simulink model "ai_optimal_path_depth_v2_3_g100"  (R2020a)
settings: Solver=FixedStepDiscrete  StartTime=0.0  StopTime=inf  FixedStep=0.2  RelTol=1e-3  EnableMultiTasking=on
model workspace (MAT data in the model file):
  SL_ROS_VariableLengthArrays_MaxSizes.CommonInfo.ArrayTruncateAction = 'EmitWarning'
  SL_ROS_VariableLengthArrays_MaxSizes.MsgTypeMap = containers.Map
  SL_ROS_VariableLengthArrays_MaxSizes.MsgTypeMap.serialization.keys = {'sensor_msgs/LaserScan', 'sensor_msgs/PointCloud2', 'std_msgs/Float64MultiArray'}
  SL_ROS_VariableLengthArrays_MaxSizes.MsgTypeMap.serialization.values{1}(1).PropertyName = 'Intensities'
  SL_ROS_VariableLengthArrays_MaxSizes.MsgTypeMap.serialization.values{1}(1).DataType = 'single'
  SL_ROS_VariableLengthArrays_MaxSizes.MsgTypeMap.serialization.values{1}(1).MaxLength = 360
  SL_ROS_VariableLengthArrays_MaxSizes.MsgTypeMap.serialization.values{1}(2).PropertyName = 'Ranges'
  SL_ROS_VariableLengthArrays_MaxSizes.MsgTypeMap.serialization.values{1}(2).DataType = 'single'
  SL_ROS_VariableLengthArrays_MaxSizes.MsgTypeMap.serialization.values{1}(2).MaxLength = 360
  SL_ROS_VariableLengthArrays_MaxSizes.MsgTypeMap.serialization.values{2}(1).PropertyName = 'Data'
  SL_ROS_VariableLengthArrays_MaxSizes.MsgTypeMap.serialization.values{2}(1).DataType = 'uint8'
  SL_ROS_VariableLengthArrays_MaxSizes.MsgTypeMap.serialization.values{2}(1).MaxLength = 600000
  SL_ROS_VariableLengthArrays_MaxSizes.MsgTypeMap.serialization.values{2}(2).PropertyName = 'Fields'
  SL_ROS_VariableLengthArrays_MaxSizes.MsgTypeMap.serialization.values{2}(2).DataType = 'sensor_msgs/PointField'
  SL_ROS_VariableLengthArrays_MaxSizes.MsgTypeMap.serialization.values{2}(2).MaxLength = 16
  SL_ROS_VariableLengthArrays_MaxSizes.MsgTypeMap.serialization.values{3}.PropertyName = 'Data'
  SL_ROS_VariableLengthArrays_MaxSizes.MsgTypeMap.serialization.values{3}.DataType = 'double'
  SL_ROS_VariableLengthArrays_MaxSizes.MsgTypeMap.serialization.values{3}.MaxLength = 360
  SL_ROS_VariableLengthArrays_MaxSizes.MsgTypeMap.serialization.uniformity = 0
  SL_ROS_VariableLengthArrays_MaxSizes.MsgTypeMap.serialization.keyType = 'char'
  SL_ROS_VariableLengthArrays_MaxSizes.MsgTypeMap.serialization.valueType = 'any'
undefined symbols (not defined in the file): Data, Data_SL_Info
libraries: robotlib x29
(part 1 of 2)
settings Model: Creator=USER  LastModifiedBy=USER
settings SolverCC: InsertRTBMode=Never (minimum delay)
settings DataIOCC: ReturnWorkspaceOutputs=off
settings OptimizationCC: StrengthReduction=on  PassReuseOutputArgsAs=Individual arguments  MaxStackSize=64  OptimizeBlockOrder=speed  OptimizationPriority=Speed  OptimizationCustomize=off  MultiThreadedLoops=on  EfficientTunableParamExpr=on
settings DebuggingCC: ParameterTunabilityLossMsg=error  PregeneratedLibrarySubsystemCodeDiagnostic=none  ArithmeticOperatorsInVariantConditions=warning
settings HardwareCC: ProdBitPerPointer=32  ProdBitPerSizeT=32  ProdBitPerPtrDiffT=32  ProdLargestAtomicFloat=None  ProdIntDivRoundTo=Undefined  ProdEndianess=Unspecified  ProdWordSize=32  ProdHWDeviceType=Generic->Unspecified (assume 32-bit Generic)
settings SFSimCC: SimUseLocalCustomCode=off  MATLABDynamicMemAlloc=off  CustomCodeUndefinedFunction=UseInterfaceOnly
settings RTWCC: SystemTargetFile=ert.tlc  HardwareBoard=Robot Operating System (ROS)  TemplateMakefile=ert_default_tmf  GenerateReport=on  RTWUseLocalCustomCode=off  Toolchain=Catkin  BuildConfiguration=Faster Runs  IncludeHyperlinkInReport=on  LaunchReport=on  TargetLang=C++  GenerateTraceInfo=on  GenerateTraceReport=on  GenerateTraceReportSl=on  GenerateTraceReportSf=on  GenerateTraceReportEml=on
settings CodeAppCC: ForceParamTrailComments=on  IgnoreCustomStorageClasses=off  OperatorAnnotations=on  SimulinkDataObjDesc=on  SFDataObjDesc=on  InsertBlockDesc=on
settings ERTTargetCC: SupportVariableSizeSignals=on

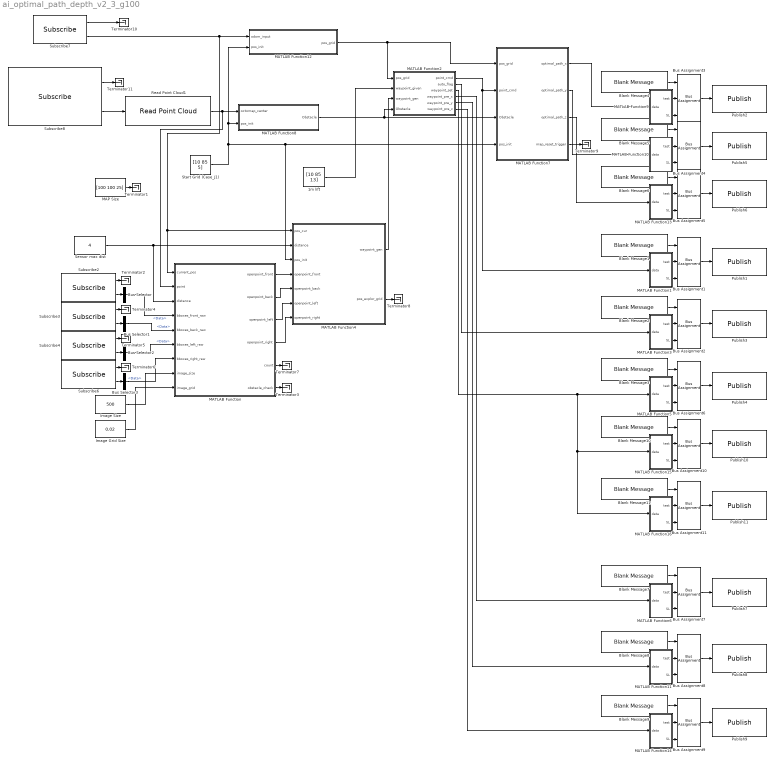
== system ai_optimal_path_depth_v2_3_g100 ==
  1m lift : Constant  Value=[10 85 13]  VectorParams1D=off
  Blank Message{1..11} (11 alike) : robotlib/Blank Message  messageClass=Message  entityType=std_msgs/Float32MultiArray  messageType=std_msgs/Float32MultiArray  SampleTime=-1
  Bus Assignment{1..11} (11 alike) : BusAssignment  AssignedSignals=Data,Data_SL_Info.CurrentLength
  Bus Selector{,1..3} (4 alike) : BusSelector  OutputSignals=Data
  Image Grid Size : Constant  Value=0.02
  Image Size : Constant  Value=500
  MAP Size : Constant  Value=[100 100 25]
  MATLAB Function : MATLAB Function  TreatAsAtomicUnit=on
  MATLAB Function1 : MATLAB Function  TreatAsAtomicUnit=on
  MATLAB Function10 : MATLAB Function  TreatAsAtomicUnit=on
  MATLAB Function11 : MATLAB Function  TreatAsAtomicUnit=on
  MATLAB Function12 : MATLAB Function  TreatAsAtomicUnit=on
  MATLAB Function13 : MATLAB Function  TreatAsAtomicUnit=on
  MATLAB Function14 : MATLAB Function  TreatAsAtomicUnit=on
  MATLAB Function15 : MATLAB Function  TreatAsAtomicUnit=on
  MATLAB Function16 : MATLAB Function  TreatAsAtomicUnit=on
  MATLAB Function2 : MATLAB Function  TreatAsAtomicUnit=on
  MATLAB Function3 : MATLAB Function  TreatAsAtomicUnit=on
  MATLAB Function4 : MATLAB Function  TreatAsAtomicUnit=on
  MATLAB Function5 : MATLAB Function  TreatAsAtomicUnit=on
  MATLAB Function6 : MATLAB Function  TreatAsAtomicUnit=on
  MATLAB Function7 : MATLAB Function  TreatAsAtomicUnit=on
  MATLAB Function8 : MATLAB Function  TreatAsAtomicUnit=on
  MATLAB Function9 : MATLAB Function  TreatAsAtomicUnit=on
  Publish1 : robotlib/Publish  topicSource=Specify your own  topic=/current_point_cmd  messageType=std_msgs/Float32MultiArray  messageQueueLength=1
  Publish10 : robotlib/Publish  topicSource=Specify your own  topic=/waypoint_set_y  messageType=std_msgs/Float32MultiArray  messageQueueLength=1
  Publish11 : robotlib/Publish  topicSource=Specify your own  topic=/waypoint_set_z  messageType=std_msgs/Float32MultiArray  messageQueueLength=1
  Publish2 : robotlib/Publish  topicSource=Specify your own  topic=/optimal_path_x  messageType=std_msgs/Float32MultiArray  messageQueueLength=1
  Publish3 : robotlib/Publish  topicSource=Specify your own  topic=/auto_flag  messageType=std_msgs/Float32MultiArray  messageQueueLength=1
  Publish4 : robotlib/Publish  topicSource=Specify your own  topic=/waypoint_set_x  messageType=std_msgs/Float32MultiArray  messageQueueLength=1
  Publish5 : robotlib/Publish  topicSource=Specify your own  topic=/optimal_path_y  messageType=std_msgs/Float32MultiArray  messageQueueLength=1
  Publish6 : robotlib/Publish  topicSource=Specify your own  topic=/optimal_path_z  messageType=std_msgs/Float32MultiArray  messageQueueLength=1
  Publish7 : robotlib/Publish  topicSource=Specify your own  topic=/waypoint_pre_x  messageType=std_msgs/Float32MultiArray  messageQueueLength=1
  Publish8 : robotlib/Publish  topicSource=Specify your own  topic=/waypoint_pre_y  messageType=std_msgs/Float32MultiArray  messageQueueLength=1
  Publish9 : robotlib/Publish  topicSource=Specify your own  topic=/waypoint_pre_z  messageType=std_msgs/Float32MultiArray  messageQueueLength=1
  Read Point Cloud1 : robotlib/Read Point Cloud  MaximumPointCloudSize=[1, 650000]  PreserveStructure=off  ShowRGBOutput=off  ShowIntensityOutput=off  ShowErrorCodeOutput=off  VariableSizeOutputs=on
      settings: SourceProductBaseCode=RR
  Sensor max dist : Constant  Value=4
  Start Grid (Case_J1) : Constant  Value=[10 85 5]
  Subscribe2 : robotlib/Subscribe  topicSource=Select from ROS network  topic=/bboxes_front  messageType=std_msgs/Float32MultiArray  sampleTime=-1  messageQueueLength=1
  Subscribe3 : robotlib/Subscribe  topicSource=Select from ROS network  topic=/bboxes_back  messageType=std_msgs/Float32MultiArray  sampleTime=-1  messageQueueLength=1
  Subscribe4 : robotlib/Subscribe  topicSource=Select from ROS network  topic=/bboxes_left  messageType=std_msgs/Float32MultiArray  sampleTime=-1  messageQueueLength=1
  Subscribe6 : robotlib/Subscribe  topicSource=Select from ROS network  topic=/bboxes_right  messageType=std_msgs/Float32MultiArray  sampleTime=-1  messageQueueLength=1
  Subscribe7 : robotlib/Subscribe  topicSource=Select from ROS network  topic=/rtabmap/odom  messageType=nav_msgs/Odometry  sampleTime=-1  messageQueueLength=1
  Subscribe8 : robotlib/Subscribe  topicSource=Select from ROS network  topic=/rtabmap/cloud_map  messageType=sensor_msgs/PointCloud2  sampleTime=-1  messageQueueLength=1
  Terminator{1..11} (11 alike) : Terminator
  wires:
  MATLAB Function9/1(test) -> Bus Assignment3/2
  Blank Message4/1 -> Bus Assignment3/1
  Bus Assignment4/1 -> Publish5/1
  Blank Message5/1 -> Bus Assignment4/1
  MATLAB Function9/2(SL) -> Bus Assignment3/3
  Subscribe7/2 -> MATLAB Function4/1(pos_cur), MATLAB Function/1(current_pos), MATLAB Function12/1(odom_input)
  MATLAB Function13/2(SL) -> Bus Assignment5/3
  Start Grid (Case_J1)/1 -> MATLAB Function4/3(pos_init), MATLAB Function7/4(pos_init), MATLAB Function8/2(pos_init), MATLAB Function12/2(pos_init)
  MATLAB Function12/1(pos_grid) -> MATLAB Function7/1(pos_grid), MATLAB Function2/1(pos_grid)
  MATLAB Function10/1(test) -> Bus Assignment4/2
  MATLAB Function13/1(test) -> Bus Assignment5/2
  Bus Assignment5/1 -> Publish6/1
  MATLAB Function10/2(SL) -> Bus Assignment4/3
  Blank Message6/1 -> Bus Assignment5/1
  Bus Assignment3/1 -> Publish2/1
  MAP Size/1 -> Terminator1/1
  MATLAB Function8/1(Obstacle) -> MATLAB Function7/3(Obstacle), MATLAB Function2/4(Obstacle)
  MATLAB Function7/1(optimal_path_x) -> MATLAB Function9/1(data)
  MATLAB Function7/2(optimal_path_y) -> MATLAB Function10/1(data)
  MATLAB Function7/3(optimal_path_z) -> MATLAB Function13/1(data)
  1m lift/1 -> MATLAB Function2/2(waypoint_given)
  Read Point Cloud1/1 -> MATLAB Function/2(point), MATLAB Function8/1(octomap_center)
  Subscribe8/2 -> Read Point Cloud1/1
  MATLAB Function2/1(point_cmd) -> MATLAB Function7/2(point_cmd), MATLAB Function1/1(data)
  Subscribe2/1 -> Terminator2/1
  Subscribe3/1 -> Terminator4/1
  Subscribe4/1 -> Terminator5/1
  Subscribe6/1 -> Terminator6/1
  Subscribe2/2 -> Bus Selector/1
  Subscribe3/2 -> Bus Selector1/1
  Subscribe4/2 -> Bus Selector2/1
  Subscribe6/2 -> Bus Selector3/1
  Image Size/1 -> MATLAB Function/8(image_size)
  Image Grid Size/1 -> MATLAB Function/9(image_grid)
  Sensor max dist/1 -> MATLAB Function4/2(distance), MATLAB Function/3(distance)
  MATLAB Function/1(openpoint_front) -> MATLAB Function4/4(openpoint_front)
  MATLAB Function/2(openpoint_back) -> MATLAB Function4/5(openpoint_back)
  MATLAB Function/3(openpoint_left) -> MATLAB Function4/6(openpoint_left)
  MATLAB Function/4(openpoint_right) -> MATLAB Function4/7(openpoint_right)
  MATLAB Function/5(count) -> Terminator7/1
  MATLAB Function4/2(pos_explor_grid) -> Terminator8/1
  Bus Selector/1 -> MATLAB Function/4(bboxes_front_raw)  "<Data>"
  Bus Selector1/1 -> MATLAB Function/5(bboxes_back_raw)  "<Data>"
  Bus Selector2/1 -> MATLAB Function/6(bboxes_left_raw)  "<Data>"
  Bus Selector3/1 -> MATLAB Function/7(bboxes_right_raw)  "<Data>"
  MATLAB Function7/4(map_reset_trigger) -> Terminator9/1
  MATLAB Function4/1(waypoint_gen) -> MATLAB Function2/3(waypoint_gen)
  MATLAB Function2/2(auto_flag) -> MATLAB Function3/1(data)
  MATLAB Function2/3(waypoint_set) -> MATLAB Function16/1(data), MATLAB Function15/1(data), MATLAB Function5/1(data)
  MATLAB Function1/1(test) -> Bus Assignment1/2
  Bus Assignment1/1 -> Publish1/1
  MATLAB Function1/2(SL) -> Bus Assignment1/3
  Blank Message1/1 -> Bus Assignment1/1
  Blank Message2/1 -> Bus Assignment2/1
  MATLAB Function3/2(SL) -> Bus Assignment2/3
  MATLAB Function3/1(test) -> Bus Assignment2/2
  Bus Assignment2/1 -> Publish3/1
  Blank Message3/1 -> Bus Assignment6/1
  MATLAB Function5/2(SL) -> Bus Assignment6/3
  MATLAB Function5/1(test) -> Bus Assignment6/2
  Bus Assignment6/1 -> Publish4/1
  MATLAB Function6/2(SL) -> Bus Assignment7/3
  MATLAB Function6/1(test) -> Bus Assignment7/2
  Blank Message7/1 -> Bus Assignment7/1
  Bus Assignment7/1 -> Publish7/1
  MATLAB Function11/1(test) -> Bus Assignment8/2
  Bus Assignment8/1 -> Publish8/1
  MATLAB Function11/2(SL) -> Bus Assignment8/3
  Blank Message8/1 -> Bus Assignment8/1
  MATLAB Function14/1(test) -> Bus Assignment9/2
  Bus Assignment9/1 -> Publish9/1
  MATLAB Function14/2(SL) -> Bus Assignment9/3
  Blank Message9/1 -> Bus Assignment9/1
  MATLAB Function2/4(waypoint_pre_x) -> MATLAB Function6/1(data)
  MATLAB Function2/5(waypoint_pre_y) -> MATLAB Function11/1(data)
  MATLAB Function2/6(waypoint_pre_z) -> MATLAB Function14/1(data)
  Subscribe7/1 -> Terminator10/1
  Subscribe8/1 -> Terminator11/1
  MATLAB Function15/1(test) -> Bus Assignment10/2
  Blank Message10/1 -> Bus Assignment10/1
  MATLAB Function15/2(SL) -> Bus Assignment10/3
  Bus Assignment10/1 -> Publish10/1
  MATLAB Function16/1(test) -> Bus Assignment11/2
  Blank Message11/1 -> Bus Assignment11/1
  MATLAB Function16/2(SL) -> Bus Assignment11/3
  Bus Assignment11/1 -> Publish11/1
  MATLAB Function/6(obstacle_check) -> Terminator3/1

== matlab function ai_optimal_path_depth_v2_3_g100/MATLAB Function10 ==
  data: data input size=[128 1]; test output size=[1 128]; SL output
function [test,SL]   = func(data)

% test = single(nan(1,128));

test = data';
% for i = 1:length(data)
%     test(i) = single(data(i));
% end

SL = uint32(length(data));


end

== matlab function ai_optimal_path_depth_v2_3_g100/MATLAB Function11 ==
  data: data input size=[20 1]; test output size=[1 128]; SL output
function [test,SL]   = func(data)

% test = single(nan(1,128));

test = single([data(:,1)', nan(1,108)]);
% for i = 1:length(data)
%     test(i) = single(data(i));
% end

SL = uint32(length(data(:,1)));


end

== matlab function ai_optimal_path_depth_v2_3_g100/MATLAB Function12 ==
  data: odom_input input; pos_grid output; pos_init input
function pos_grid = odom_grid(odom_input,pos_init)

odom = zeros(1,3);


% odom(1,1) = odom_input.Poses(end).Pose.Position.X;
% odom(1,2) = odom_input.Poses(end).Pose.Position.Y;
% odom(1,3) = odom_input.Poses(end).Pose.Position.Z;

odom(1,1) = odom_input.Pose.Pose.Position.X;
odom(1,2) = odom_input.Pose.Pose.Position.Y;
odom(1,3) = odom_input.Pose.Pose.Position.Z;

start_point = [pos_init(1) pos_init(2) pos_init(3)];

% pos_x = int16(odom(1)/0.2+0.5);
% pos_y = int16(odom(2)/0.2+0.5);
% pos_z = int16(odom(3)/0.2+0.5);
pos_x = int16(odom(1)/0.1);
pos_y = int16(odom(2)/0.1);
pos_z = int16(odom(3)/0.1);

pos_grid = [pos_x+start_point(1) pos_y+start_point(2) pos_z+start_point(3)];


end

== matlab function ai_optimal_path_depth_v2_3_g100/MATLAB Function13 ==
  data: data input size=[128 1]; test output size=[1 128]; SL output
function [test,SL]   = func(data)


% test = single(nan(1,128));

test = data';
% for i = 1:length(data)
%     test(i) = single(data(i));
% end

SL = uint32(length(data));

end

== matlab function ai_optimal_path_depth_v2_3_g100/MATLAB Function7 ==
  data: pos_grid input; optimal_path_x output size=[128 1]; point_cmd input; Obstacle input; pos_init input; optimal_path_y output size=[128 1]; optimal_path_z output size=[128 1]; map_reset_trigger output
function [optimal_path_x,optimal_path_y,optimal_path_z,map_reset_trigger] = Astar_algorithm_function(pos_grid,point_cmd,Obstacle,pos_init)

    persistent optimal astar_restart curr_point hover_flag 

    if isempty(optimal)
        optimal = nan(128,3);
        hover_flag = 0;
        astar_restart = 1;
        curr_point = point_cmd;        
    end

    map_reset_trigger = 0;
    grid_size = 0.1;

    if (curr_point(1) ~= point_cmd(1)) || (curr_point(2) ~= point_cmd(2)) || (curr_point(3) ~= point_cmd(3))
        astar_restart = 1;
    end
    curr_point = point_cmd;
    
    if Obstacle(pos_grid(1), pos_grid(2), pos_grid(3)) == 1
        astar_restart = 0;
    end
    
    
%---------------------------------------------------------
% A* 시작
%---------------------------------------------------------
    if astar_restart == 1
        % ----------------------------------------------------- initilize
        astar_restart = 0;
        mapsize = [140 120 30];
        
        Height = mapsize(1);        % x
        Width = mapsize(2);         % y
        Alt = mapsize(3);            % z
        
        Start = pos_grid;
%         Goal = int32(point_cmd/grid_size + pos_init');          % 수정 
        Goal = int32(point_cmd);          % 수정 
        look = 2;
        H_weight = 1.3;
        
        G_cost = zeros(2*look+1,2*look+1,2*look+1);
        for i = 1:2*look+1
            for j = 1:2*look+1
                for k = 1:2*look+1
                    temp = [look+1 look+1 look+1]-[i j k];
                    G_cost(i,j,k) = (min(sqrt(sum(abs(temp).^2,2))));
                end
            end
        end
        
        G_top2 = G_cost(:,:,1);
        G_top1 = G_cost(:,:,2);
        G_mid = G_cost(:,:,3);
        G_bottom1 = G_cost(:,:,4);
        G_bottom2 = G_cost(:,:,5);
        
        
        GScore = inf(Height,Width,Alt);
        GScore_temp = zeros(2*look+1,2*look+1,2*look+1);
        HScore = zeros(Height,Width,Alt);
        FScore = inf(Height,Width,Alt);
        ClosedMAT = zeros(Height,Width,Alt);
        CX = int32(Start(1));
        CY = int32(Start(2));
        CZ = int32(Start(3));
        ParentX = inf(Height,Width,Alt);
        ParentY = inf(Height,Width,Alt);
        ParentZ = inf(Height,Width,Alt);
        ParentX(CX,CY,CZ) = CX;
        ParentY(CX,CY,CZ) = CY;
        ParentZ(CX,CY,CZ) = CZ;
        hover_flag = 0;
        
        %%%%%%%%%%%%%%%% Define Heuristic %%%%%%%%%%%%%%%%%%%%%%%
        for k=1:Alt
            for j=1:Width
                for i=1:Height
                    
                    temp = (int32(Goal) - int32([i j k])) ;
                    Distance=(min(sqrt(sum(abs(temp).^2,2))));
                    HScore(i,j,k)=Distance*H_weight;               % (1+sqrt(2))/sqrt(3)
                    
                end
            end
        end
        
        FScore(Start(1),Start(2),Start(3)) = HScore(Start(1),Start(2),Start(3));
        GScore(Start(1),Start(2),Start(3)) = 0;
        ClosedMAT(Obstacle==1)=1;
        REACHGOAL = 0;
        
        while 1
            fprintf("A* loop \n");
            MinFScore = min(min(min(FScore)));         % Find Minimun FScore
            
            if isinf(MinFScore)
                hover_flag = 1;
                astar_restart = 1;
                map_reset_trigger = 1;
                fprintf("No path -> restart A*, Map reset \n");
                break
            end
            
            [minF_x,minF_y] = find(FScore==MinFScore);
            HScore_temp = inf(1,10);
            
            minHScore = 1;
            for i = 1:length(minF_x)
                Current_pose_temp = [minF_x(i) rem(minF_y(i),Width) fix(minF_y(i)/Width)+1];     % H가 가장 적은걸로 먼저 선택
                CX_temp=Current_pose_temp(1);
                CY_temp=Current_pose_temp(2);
                CZ_temp=Current_pose_temp(3);
                HScore_temp(i) = HScore(CX_temp,CY_temp,CZ_temp);
                minHScore = find(HScore_temp == min(HScore_temp));
            end
            
            Current_pose = int32([minF_x(minHScore(1)) rem(minF_y(minHScore(1)),Width) fix(minF_y(minHScore(1))/Width)+1]);     % H가 가장 적은걸로 먼저 선택
            CX=Current_pose(1);
            CY=Current_pose(2);
            CZ=Current_pose(3);

            GScore_temp(:,:,1) = GScore(CX,CY,CZ) + G_top2;
            GScore_temp(:,:,2) = GScore(CX,CY,CZ) + G_top1;
            GScore_temp(:,:,3) = GScore(CX,CY,CZ) + G_mid;
            GScore_temp(:,:,4) = GScore(CX,CY,CZ) + G_bottom1;
            GScore_temp(:,:,5) = GScore(CX,CY,CZ) + G_bottom2;
            
            %%%%%%%%%%%%% GScore update %%%%%%%%%%%%%
            GScore(CX-look:CX+look,CY-look:CY+look,CZ+2) = min(GScore_temp(:,:,1),GScore(CX-look:CX+look,CY-look:CY+look,CZ+2)) ;
            GScore(CX-look:CX+look,CY-look:CY+look,CZ+1) = min(GScore_temp(:,:,2),GScore(CX-look:CX+look,CY-look:CY+look,CZ+1));
            GScore(CX-look:CX+look,CY-look:CY+look,CZ) = min(GScore_temp(:,:,3), GScore(CX-look:CX+look,CY-look:CY+look,CZ));
            GScore(CX-look:CX+look,CY-look:CY+look,CZ-1) = min(GScore_temp(:,:,4),GScore(CX-look:CX+look,CY-look:CY+look,CZ-1));
            GScore(CX-look:CX+look,CY-look:CY+look,CZ-2) = min(GScore_temp(:,:,5),GScore(CX-look:CX+look,CY-look:CY+look,CZ-2));
            
            FScore = GScore + HScore;
            ClosedMAT(CX-(look-1):CX+(look-1),CY-(look-1):CY+(look-1),CZ-(look-1):CZ+(look-1)) = 1;
            FScore(ClosedMAT==1) = inf;
            
            [G_row1,G_col1] = find( GScore(CX-look:CX+look,CY-look:CY+look,CZ+2) == GScore_temp(:,:,1) );
            [G_row2,G_col2] = find( GScore(CX-look:CX+look,CY-look:CY+look,CZ+1) == GScore_temp(:,:,2) );
            [G_row3,G_col3] = find( GScore(CX-look:CX+look,CY-look:CY+look,CZ) == GScore_temp(:,:,3) );
            [G_row4,G_col4] = find( GScore(CX-look:CX+look,CY-look:CY+look,CZ-1) == GScore_temp(:,:,4) );
            [G_row5,G_col5] = find( GScore(CX-look:CX+look,CY-look:CY+look,CZ-2) == GScore_temp(:,:,5) );
            
            G_row1 = int32(G_row1);
            G_row2 = int32(G_row2);
            G_row3 = int32(G_row3);
            G_row4 = int32(G_row4);
            G_row5 = int32(G_row5);
            
            G_col1 = int32(G_col1);
            G_col2 = int32(G_col2);
            G_col3 = int32(G_col3);
            G_col4 = int32(G_col4);
            G_col5 = int32(G_col5);
            
            G_row1 = G_row1+CX-(look+1);
            G_row2 = G_row2+CX-(look+1);
            G_row3 = G_row3+CX-(look+1);
            G_row4 = G_row4+CX-(look+1);
            G_row5 = G_row5+CX-(look+1);
            
            G_col1 = G_col1+CY-(look+1);
            G_col2 = G_col2+CY-(look+1);
            G_col3 = G_col3+CY-(look+1);
            G_col4 = G_col4+CY-(look+1);
            G_col5 = G_col5+CY-(look+1);
            
            for i = 1:length(G_row1)
                ParentX(G_row1(i),G_col1(i),CZ+2) = CX;
                ParentY(G_row1(i),G_col1(i),CZ+2) = CY;
                ParentZ(G_row1(i),G_col1(i),CZ+2) = CZ;
            end
            
            for i = 1:length(G_row2)
                ParentX(G_row2(i),G_col2(i),CZ+1) = CX;
                ParentY(G_row2(i),G_col2(i),CZ+1) = CY;
                ParentZ(G_row2(i),G_col2(i),CZ+1) = CZ;
            end
            
            for i = 1:length(G_row3)
                if G_row3(i)==CX && G_col3(i)==CY
                    continue
                end
                ParentX(G_row3(i),G_col3(i),CZ) = CX;
                ParentY(G_row3(i),G_col3(i),CZ) = CY;
                ParentZ(G_row3(i),G_col3(i),CZ) = CZ;
            end
            
            for i = 1:length(G_row4)
                ParentX(G_row4(i),G_col4(i),CZ-1) = CX;
                ParentY(G_row4(i),G_col4(i),CZ-1) = CY;
                ParentZ(G_row4(i),G_col4(i),CZ-1) = CZ;
            end
            
            for i = 1:length(G_row5)
                ParentX(G_row5(i),G_col5(i),CZ-2) = CX;
                ParentY(G_row5(i),G_col5(i),CZ-2) = CY;
                ParentZ(G_row5(i),G_col5(i),CZ-2) = CZ;
            end
            
            if abs(Goal(1)-CX)<=(look-1) && abs(Goal(2)-CY)<=(look-1) && abs(Goal(3)-CZ)<=(look-1)
                REACHGOAL = 1;
                fprintf("path founded\n");
                break
            end
        end
        
        optimal = nan(128,3);
        if REACHGOAL
            optimal(1,:) = [Goal(1) Goal(2) Goal(3)];
            k=2;
            while 1
                CX_temp = int32(ParentX(CX,CY,CZ));
                CY_temp = int32(ParentY(CX,CY,CZ));
                CZ_temp = int32(ParentZ(CX,CY,CZ));
                
                CX = CX_temp;
                CY = CY_temp;
                CZ = CZ_temp;
                
                optimal(k,:) = [CX CY CZ];
                k = k+1;
                
                if CX==Start(1) && CY==Start(2) && CZ==Start(3)
                    break
                end
            end
        end
        
    end
    
    if hover_flag == 0
            nan_check = isnan(optimal(:,1));
            for i = 1:1:128
                if nan_check(i) == 0
                    %fprintf("i:%d (%d,%d,%d) %d    ", int32(i), int32(optimal(i,1)), int32(optimal(i,2)), int32(optimal(i,3)), int32(Obstacle(optimal(i,1), optimal(i,2), optimal(i,3))));
                    if Obstacle(optimal(i,1), optimal(i,2), optimal(i,3)) == 1
                        astar_restart = 1;
                        fprintf("path collision! \n");
                        break;
                    end
                    %fprintf("not break \n");
                end
                astar_restart = 0;
            end
            % fprintf("collision check done \n");
    end
        
    if hover_flag == 1
        fprintf("hover flag on \n");
        hover_point = nan(128,3);
        hover_point(1,:) = [pos_grid(1) pos_grid(2) pos_grid(3)];
        optimal_path_x = flip(single( (hover_point(:,1)-pos_init(1)) * grid_size ));      % grid_size = 0.2,
        optimal_path_y = flip(single( (hover_point(:,2)-pos_init(2)) * grid_size ));
        optimal_path_z = flip(single( (hover_point(:,3)-pos_init(3)) * grid_size ));
    else
        optimal_path_x = flip(single( (optimal(:,1)-pos_init(1)) * grid_size ));      % grid_size = 0.2
        optimal_path_y = flip(single( (optimal(:,2)-pos_init(2)) * grid_size ));
        optimal_path_z = flip(single( (optimal(:,3)-pos_init(3)) * grid_size ));
    end
    
    
end

== matlab function ai_optimal_path_depth_v2_3_g100/MATLAB Function8 ==
  data: octomap_center input size=[650000 3]; Obstacle output size=[140 120 30]; pos_init input
function Obstacle = gen_3d_array(octomap_center,pos_init)
mapsize=[140 120 30];
Obstacle = int8(zeros(mapsize(1),mapsize(2),mapsize(3)));
start_point = [pos_init(1) pos_init(2) pos_init(3)];

grid_size = 0.1;
drone_size_xy = 0.2; % m
safety_size_xy = 0.2; % m
drone_size_z = 0.1; % m
safety_size_z = 0.1; % m
scattering_cells_xy = ceil((drone_size_xy + safety_size_xy)/grid_size);
scattering_cells_z = ceil((drone_size_z + safety_size_z)/grid_size);

test=[scattering_cells_xy+1 scattering_cells_xy+1 scattering_cells_z+1];

scattering_array = int8(zeros(scattering_cells_xy*2+1, scattering_cells_xy*2+1, scattering_cells_z*2+1));
for i=0:scattering_cells_xy
    for j=0:scattering_cells_xy
        if i^2+j^2 <= ((drone_size_xy + safety_size_xy)/grid_size)^2 
            scattering_array(i+test(1), j+test(2), -scattering_cells_z+test(3):scattering_cells_z + test(3)) = 1;
            scattering_array(i+test(1), -j+test(2), -scattering_cells_z+test(3):scattering_cells_z + test(3)) = 1;
            scattering_array(-i+test(1), j+test(2), -scattering_cells_z+test(3):scattering_cells_z + test(3)) = 1;
            scattering_array(-i+test(1), -j+test(2), -scattering_cells_z+test(3):scattering_cells_z + test(3)) = 1;
        end
    end
end
% scattering_array

align1 = int16(octomap_center/(grid_size));
align2 = unique(align1,'rows');
align3 = [align2(:,1)+start_point(1) align2(:,2)+start_point(2) align2(:,3)+start_point(3)]; % for ROS axis
%align3 = [align2(:,2)+start_point(1) -align2(:,1)+start_point(2) align2(:,3)+start_point(3)]; % for Fiesta axis

for i = 1:numel(align3)/3
    
    index_temp = align3(i,:);

    for j=1:scattering_cells_xy*2+1
        if index_temp(1)+j-1 - scattering_cells_xy <= 0 || index_temp(1)+j-1 - scattering_cells_xy > mapsize(1)
            continue;
        end    
        for k=1:scattering_cells_xy*2+1
            if index_temp(2)+k-1 -scattering_cells_xy <= 0 || index_temp(2)+k-1 - scattering_cells_xy > mapsize(2)
                continue;
            end
            for l=1:scattering_cells_z*2+1
                if index_temp(3)+l-1 - scattering_cells_z <= 0 || index_temp(3)+l-1 - scattering_cells_z > mapsize(3)
                    continue;
                end
                if scattering_array(j, k, l) == 1
                    Obstacle(index_temp(1)+j-1-scattering_cells_xy, index_temp(2)+k-1-scattering_cells_xy, index_temp(3)+l-1-scattering_cells_z) = 1;
                end
            end

        end
    end
end

Obstacle(1:3,:,:)=1;
Obstacle(mapsize(1)-2:mapsize(1),:,:) = 1;
Obstacle(:,1:3,:) = 1;
Obstacle(:,mapsize(2)-2:mapsize(2),:) = 1;
Obstacle(:,:,1:4) = 1;
Obstacle(:,:,mapsize(3)-10:mapsize(3)) = 1; % 고도제한 1.5m 

end

== matlab function ai_optimal_path_depth_v2_3_g100/MATLAB Function9 ==
  data: data input size=[128 1]; test output size=[1 128]; SL output
function [test,SL]   = func(data)

% test = single(nan(1,128));

test = data';
% for i = 1:length(data)
%     test(i) = single(data(i));
% end

SL = uint32(length(data));


end

== matlab function ai_optimal_path_depth_v2_3_g100/MATLAB Function14 ==
  data: data input size=[20 1]; test output size=[1 128]; SL output
function [test,SL]   = func(data)

% test = single(nan(1,128));

test = single([data(:,1)', nan(1,108)]);
% for i = 1:length(data)
%     test(i) = single(data(i));
% end

SL = uint32(length(data(:,1)));


end

== matlab function ai_optimal_path_depth_v2_3_g100/MATLAB Function15 ==
  data: data input size=[40 3]; test output size=[1 128]; SL output
function [test,SL]   = func(data)

% test = single(nan(1,128));

test = single([data(:,2)', nan(1,88)]);
% for i = 1:length(data)
%     test(i) = single(data(i));
% end

SL = uint32(length(data(:,2)));


end

== matlab function ai_optimal_path_depth_v2_3_g100/MATLAB Function16 ==
  data: data input size=[40 3]; test output size=[1 128]; SL output
function [test,SL]   = func(data)

% test = single(nan(1,128));

test = single([data(:,3)', nan(1,88)]);
% for i = 1:length(data)
%     test(i) = single(data(i));
% end

SL = uint32(length(data(:,3)));


end

== matlab function ai_optimal_path_depth_v2_3_g100/MATLAB Function1 ==
  data: data input size=[1 3]; test output size=[1 128]; SL output
function [test,SL]   = func(data)
% function [test,SL]   = func(data,pos_init)

% test = single(nan(1,128));

% test = single([single(data)-single(pos_init'), nan(1,125)])*0.2;
test = single([data, nan(1,125)]);
% for i = 1:length(data)
%     test(i) = single(data(i));
% end

SL = uint32(length(data));


end

== matlab function ai_optimal_path_depth_v2_3_g100/MATLAB Function2 ==
  data: pos_grid input; point_cmd output; waypoint_given input; waypoint_gen input; Obstacle input; auto_flag output; waypoint_set output; waypoint_pre_x output; waypoint_pre_y output; waypoint_pre_z output
function [point_cmd,auto_flag,waypoint_set,waypoint_pre_x,waypoint_pre_y,waypoint_pre_z] = gen_waypoint(pos_grid,waypoint_given,waypoint_gen,Obstacle)

persistent flag autonomous_mode_flag waypoint_old waypoint_pre

if isempty(flag)
    flag = 1;
end
if isempty(autonomous_mode_flag)
    autonomous_mode_flag = 0;
%     autonomous_mode_flag = 1;
end
if isempty(waypoint_old)
    waypoint_old = nan(20,3);
end
% num_waypoint_given = numel(waypoint_given)/3;
num_waypoint_given = 1;
if isempty(waypoint_pre)
    waypoint_pre = nan(20,3);
    for aaa = 1:num_waypoint_given
        waypoint_pre(aaa,1)=waypoint_given(aaa,1);
        waypoint_pre(aaa,2)=waypoint_given(aaa,2);
        waypoint_pre(aaa,3)=waypoint_given(aaa,3);
    end
end

pos_grid = int32(pos_grid);

waypoint_pre_x = waypoint_pre(:,1);
waypoint_pre_y = waypoint_pre(:,2);
waypoint_pre_z = waypoint_pre(:,3);

point_cmd_temp = int32([waypoint_pre_x(flag) waypoint_pre_y(flag) waypoint_pre_z(flag)]);
waypoint_gen_sorted = nan(20,3);
waypoint_auto_set = nan(40,3);
waypoint_auto_set_sorted = nan(40,3);
waypoint_distance = nan(40,1);

for lll = 1:numel(waypoint_gen)/3
    if ~isnan(waypoint_gen(lll,1)) && ~isnan(waypoint_gen(lll,2)) && ~isnan(waypoint_gen(lll,3))
        if Obstacle(waypoint_gen(lll,1),waypoint_gen(lll,2),waypoint_gen(lll,3)) == 1
            waypoint_gen(lll,:)=nan(1,3);
        end
    end
end


if autonomous_mode_flag==0
    if abs(point_cmd_temp(1)-pos_grid(1)) <= 1 && abs(point_cmd_temp(2)-pos_grid(2)) <= 1 && abs(point_cmd_temp(3)-pos_grid(3)) <= 1
        flag = flag + 1;
        
        %         if flag == numel(rmmissing(waypoint_pre))/3 + 1
        %             flag = numel(rmmissing(waypoint_pre))/3;
%         if flag == num_waypoint_given + 1
        if flag > num_waypoint_given
            flag = num_waypoint_given;
            autonomous_mode_flag = 1;
        end
    end
    
elseif autonomous_mode_flag==1
    %     waypoint_auto_old = rmmissing(waypoint_old);
    %     waypoint_auto_new = rmmissing(waypoint_gen);
    
    
    waypoint_auto_old = waypoint_old;
    [~,waypoint_gen_index]=sort(waypoint_gen(:,1));
    for aaa = 1:length(waypoint_gen_index)
        waypoint_gen_sorted(aaa,:)=waypoint_gen(waypoint_gen_index(aaa),:);
    end
    waypoint_auto_new=waypoint_gen_sorted;
%     if isempty(waypoint_auto_old)
    if sum(isnan(waypoint_auto_old),'all')==numel(waypoint_auto_old)
        waypoint_auto_old = waypoint_auto_new;
    end
    
    num_nonnan_new = 0;
    num_nonnan_old = 0;
    for ttt = 1:numel(waypoint_auto_new)/3
        if ~isnan(waypoint_auto_new(ttt,1)) && ~isnan(waypoint_auto_new(ttt,2)) && ~isnan(waypoint_auto_new(ttt,3))
            num_nonnan_new = num_nonnan_new + 1;
        end
    end
    for sss = 1:numel(waypoint_auto_old)/3
        if ~isnan(waypoint_auto_old(sss,1)) && ~isnan(waypoint_auto_old(sss,2)) && ~isnan(waypoint_auto_old(sss,3))
            num_nonnan_old = num_nonnan_old + 1;
        end
    end
    
%     if ~isempty(waypoint_auto_old) && ~isempty(waypoint_auto_new)
    if sum(isnan(waypoint_auto_old),'all')~=numel(waypoint_auto_old) && sum(isnan(waypoint_auto_new),'all')~=numel(waypoint_auto_new)
%         for mmm = numel(waypoint_auto_new)/3:-1:1
        for mmm = num_nonnan_new:-1:1
            changed_flag=0;
%             for nnn = 1:numel(waypoint_auto_old)/3
            for nnn = 1:num_nonnan_old
                if ((waypoint_auto_new(mmm,1)-waypoint_auto_old(nnn,1))^2+(waypoint_auto_new(mmm,2)-waypoint_auto_old(nnn,2))^2+(waypoint_auto_new(mmm,3)-waypoint_auto_old(nnn,3))^2)<100
                    waypoint_auto_old(nnn,:)=waypoint_auto_new(mmm,:);
                    changed_flag=1;
                end
            end
            if changed_flag == 1
                waypoint_auto_new(mmm,:)=nan(1,3);
            end
        end
%         waypoint_auto_set_temp = rmmissing(cat(1,unique(waypoint_auto_old,'stable','rows'),waypoint_auto_new));
        waypoint_auto_set_temp = cat(1,unique(waypoint_auto_old,'stable','rows'),waypoint_auto_new);
        
        
        for aaa = 1:numel(waypoint_auto_set_temp)/3
            waypoint_auto_set(aaa,:)=waypoint_auto_set_temp(aaa,:);
            waypoint_distance(aaa) = (((waypoint_auto_set(aaa,1)-pos_grid(1))^2+(waypoint_auto_set(aaa,2)-pos_grid(2))^2+(waypoint_auto_set(aaa,3)-pos_grid(3))^2));
        end
        [~,waypoint_index]=sort(waypoint_distance);
        
        for aaa = 1:length(waypoint_index)
            waypoint_auto_set_sorted(aaa,:)=waypoint_auto_set(waypoint_index(aaa),:);
        end
        
        point_cmd_temp = int32([waypoint_auto_set_sorted(1,1), waypoint_auto_set_sorted(1,2), waypoint_auto_set_sorted(1,3)]);
        
        if abs(point_cmd_temp(1)-pos_grid(1)) <= 1 && abs(point_cmd_temp(2)-pos_grid(2)) <= 1 && abs(point_cmd_temp(3)-pos_grid(3)) <= 1
            waypoint_auto_set_sorted = [waypoint_auto_set_sorted(2:end,:); nan(1,3)];
        end
        
        waypoint_old = waypoint_auto_set_sorted(1:20,:);
        
        
    else
        if ~isnan(waypoint_old(1,1)) && ~isnan(waypoint_old(1,2)) && ~isnan(waypoint_old(1,3))
            point_cmd_temp = int32([waypoint_old(1,1), waypoint_old(1,2), waypoint_old(1,3)]);
            
            if abs(point_cmd_temp(1)-pos_grid(1)) <= 1 && abs(point_cmd_temp(2)-pos_grid(2)) <= 1 && abs(point_cmd_temp(3)-pos_grid(3)) <= 1
                waypoint_old = [waypoint_old(2:end,:); nan(1,3)];
            end
            
            
        else
            point_cmd_temp = int32([pos_grid(1), pos_grid(2), pos_grid(3)]);
        end
    end
end

point_cmd = point_cmd_temp;


auto_flag = autonomous_mode_flag;
waypoint_set = waypoint_auto_set_sorted;


end

== matlab function ai_optimal_path_depth_v2_3_g100/MATLAB Function3 ==
  data: data input size=[1]; test output size=[1 128]; SL output
function [test,SL]   = func(data)

% test = single(nan(1,128));

test = single([data, nan(1,127)]);
% for i = 1:length(data)
%     test(i) = single(data(i));
% end

SL = uint32(length(data));


end
